simulink model "Caso3MultiplosPontosEquilibrio"  (R2015a)
settings: Solver=ode45  StartTime=0.0  StopTime=5e11  RelTol=1e-3
settings Model: Creator=user  LastModifiedBy=user

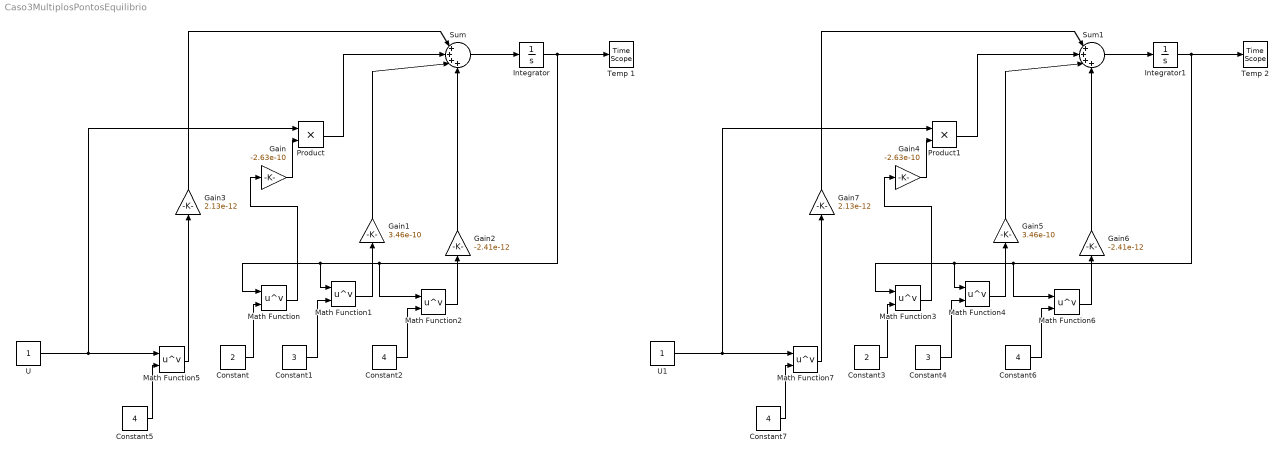
== system Caso3MultiplosPontosEquilibrio ==
  Constant : Constant  Value=2
  Constant1 : Constant  Value=3
  Constant{2,5..7} (4 alike) : Constant  Value=4
  Constant3 : Constant  Value=2
  Constant4 : Constant  Value=3
  Gain : Gain  Gain=-2.63e-10
  Gain1 : Gain  Gain=3.46e-10
  Gain2 : Gain  Gain=-2.41e-12
  Gain3 : Gain  Gain=2.13e-12
  Gain4 : Gain  Gain=-2.63e-10
  Gain5 : Gain  Gain=3.46e-10
  Gain6 : Gain  Gain=-2.41e-12
  Gain7 : Gain  Gain=2.13e-12
  Integrator : Integrator  InitialCondition=300
  Integrator1 : Integrator
  Math Function{,1..7} (8 alike) : Math  Operator=pow  SaturateOnIntegerOverflow=on
  Product : Product
  Product1 : Product
  Sum : Sum  Inputs=|++++
  Sum1 : Sum  Inputs=|++++
  Temp 1 : TimeScope
  Temp 2 : TimeScope
  U : Constant
  U1 : Constant
  wires:
  Sum/1 -> Integrator/1
  Constant/1 -> Math Function/2
  Constant1/1 -> Math Function1/2
  Constant2/1 -> Math Function2/2
  Integrator/1 -> Temp 1/1, Math Function2/1, Math Function1/1, Math Function/1
  Math Function/1 -> Gain/1
  Math Function1/1 -> Gain1/1
  Math Function2/1 -> Gain2/1
  Gain1/1 -> Sum/3
  Gain2/1 -> Sum/4
  Constant5/1 -> Math Function5/2
  Math Function5/1 -> Gain3/1
  U/1 -> Product/1, Math Function5/1
  Gain3/1 -> Sum/1
  Gain/1 -> Product/2
  Product/1 -> Sum/2
  Sum1/1 -> Integrator1/1
  Constant3/1 -> Math Function3/2
  Constant4/1 -> Math Function4/2
  Constant6/1 -> Math Function6/2
  Integrator1/1 -> Temp 2/1, Math Function6/1, Math Function4/1, Math Function3/1
  Math Function3/1 -> Gain4/1
  Math Function4/1 -> Gain5/1
  Math Function6/1 -> Gain6/1
  Gain5/1 -> Sum1/3
  Gain6/1 -> Sum1/4
  Constant7/1 -> Math Function7/2
  Math Function7/1 -> Gain7/1
  U1/1 -> Product1/1, Math Function7/1
  Gain7/1 -> Sum1/1
  Gain4/1 -> Product1/2
  Product1/1 -> Sum1/2
